simulink model "LGS_allFaultsSelected"  (R2019b)
settings: Solver=FixedStepDiscrete  StartTime=0.0  StopTime=45.0  FixedStep=0.1  RelTol=1e-3
model workspace (MAT data in the model file):
  fipData : object (value not decoded)
  fipName : object (value not decoded)
  stepSize = 0.1
undefined symbols (not defined in the file): ActualSystemCondition, ExpectedSystemBehavior, FailureCondition, FailureConditionObserver, LibFailureCondition
libraries: LibFaultInjectionControls x190, commrandsrc3 x70, simulink x3
(part 34 of 41)

== system LGS_allFaultsSelected/Gears/left gear cylinder/sensor locked retracted/FIP3/LG sensor locked retracted FIP3 ==
  In1 : Inport
  Commit Any Bool : Subsystem  mask(FailureMode){isActive=on, isDSF=off, FailureRate=1.0E-3, useDefaultMt_copy=off, MaintenanceTask=0, useDefaultMt=off, RiskTime=0, useDefaultRt=off, File=[], DSFjson=JSON}
      mask prompts: isActive "is Active"; isDSF "DSF Trigger"; useDefaultMt_copy "set"; useDefaultMt "set"; useDefaultRt "set"
      mask TypeOptions isActive: Trigger FIP/Active
      mask TypeOptions isDSF: Trigger FIP/isDSF
      mask Callback isDSF:
      | a = Simulink.Mask.get(gcb);
      | disp(a);
      | d = a.DialogControls();
      | disp(d);
      | for i = 1:size(d,2)
      |     if strcmp(d(i).Name, 'ParameterGroupVar')
      |         basicFip_ctrl = d(i).getDialogControl('BasicFipParam');
      |         dsFip_ctrl = d(i).getDialogControl('DSFipParam');
      | 
      |         if strcmp(get_param(gcb, 'isDSF'), 'on')
      | %            basicFip_ctrl.Visible = 'off';
      |             basicFip_ctrl.Enabled = 'off';
      | 
      |             dsFip_ctrl.Enabled = 'on';
      | %            dsFip_ctrl.Visible = 'on';
      |         else
      |             basicFip_ctrl.Enabled = 'on';
      | %            basicFip_ctrl.Visible = 'on';
      | 
      | %            dsFip_ctrl.Visible = 'off';
      |             dsFip_ctrl.Enabled = 'off';
      |         end
      |     end
      | end
      mask TypeOptions FailureRate: Trigger FIP/FailureRate
      mask Callback useDefaultMt_copy:
      | a = Simulink.Mask.get(gcb);
      | d = a.Parameters();
      | for i = 1:size(d,2)
      |     if strcmp(d(i).Name, 'MaintenanceTask')
      |         if strcmp(get_param(gcb, 'useDefaultMt'), 'off')
      |             set_param(gcb,'MaintenanceTask', '0')
      |             d(i).Enabled = 'off';
      |         else
      |             d(i).Enabled = 'on';
      |         end
      |     end
      | end
      mask TypeOptions MaintenanceTask: Trigger FIP/MaintenanceTask
      mask Callback useDefaultMt:
      | a = Simulink.Mask.get(gcb);
      | d = a.Parameters();
      | for i = 1:size(d,2)
      |     if strcmp(d(i).Name, 'MaintenanceTask')
      |         if strcmp(get_param(gcb, 'useDefaultMt'), 'off')
      |             set_param(gcb,'MaintenanceTask', '0')
      |             d(i).Enabled = 'off';
      |         else
      |             d(i).Enabled = 'on';
      |         end
      |     end
      | end
      mask TypeOptions RiskTime: Trigger FIP/RiskTime
      mask Callback useDefaultRt:
      | a = Simulink.Mask.get(gcb);
      | d = a.Parameters();
      | for i = 1:size(d,2)
      |     if strcmp(d(i).Name, 'RiskTime')
      |         if strcmp(get_param(gcb, 'useDefaultRt'), 'off')
      |             set_param(gcb,'RiskTime', '0')
      |             d(i).Enabled = 'off';
      |         else
      |             d(i).Enabled = 'on';
      |         end
      |     end
      | end
      mask TypeOptions DSFjson: Trigger FIP/DSFjson
      mask DialogControl DescGroupVar Prompt: Any Bool
      mask DialogControl DescTextVar Prompt: Controls for a fault with random boolean as result type
      mask DialogControl BasicFipBehavior Prompt: Failure Mode Behavior
      mask DialogControl BasicFipParamTab Prompt: Failure Mode Occurrence
      mask DialogControl BasicFipParam Prompt: Parameters
      mask DialogControl FailureRate_label Prompt: Failure Rate [1/h]
      mask DialogControl MaintenanceTask_label Prompt: Maintenance Task [h]
      mask DialogControl RiskTime_label Prompt: Risk time [h]
      mask DialogControl DSFipParamTab Prompt: Dependent System Information
      mask DialogControl DSFipParam Prompt: Parameters
      mask DialogControl LoadCSV Prompt: Browse
      mask DialogControl LoadCSV Callback:
      | [file,path,indx] = uigetfile('*.csv');
      | try
      |     set_param(gcb, 'File', append(path,file));
      |     file = fopen(append(path,file));
      | 
      |     fips = {};
      |     cutsets = {};
      | 
      |     line = fgetl(file);
      |     while ischar(line)
      |         disp(join([' > Processing: ',line]));
      |         splitString = split(line, ';');
      |         if isequal(splitString{1}, 'Cut set')
      |             disp('   > Found Cut set');
      |             cs = splitString(2:end-1);
      |             disp(cs);
      |             cutsets{end+1} = cs';
      |         else
      |             disp('   > Found FIP');
      |             if ~isequal("h", splitString(7))
      |                 disp('no time format except hour is supported');
      |             end
      |             fip = {};
      |             fip.id = splitString(1);
      |             fip.path = splitString(3);
      |             fip.rate = splitString(4);
      |             fip.checkInterval = splitString(6);
      |             disp(fip);
      |             fips{end+1} = fip;
      |         end
      |         line = fgetl(file);
      |     end
      | 
      |     fclose(file);
      | 
      |     DSF = {};
      |     DSF.fips = fips;
      |     DSF.cutsets = cutsets;
      | 
      |     VarCSText = jsonencode(DSF);
      |     set_param(gcb, 'DSFjson', VarCSText);
      | catch
      | end
  Permanently Blocked False : Subsystem  mask(FailureMode){isActive=on, isDSF=off, Value=false, FailureRate=1.0E-3, useDefaultMt_copy=off, MaintenanceTask=0, useDefaultMt=off, RiskTime=0, useDefaultRt=off, File=[], DSFjson=JSON}
      mask prompts: isActive "is Active"; isDSF "DSF Trigger"; Value "Bool Value"; useDefaultMt_copy "set"; useDefaultMt "set"; useDefaultRt "set"
      mask TypeOptions isActive: Trigger FIP/Active
      mask TypeOptions isDSF: Trigger FIP/isDSF
      mask Callback isDSF:
      | a = Simulink.Mask.get(gcb);
      | disp(a);
      | d = a.DialogControls();
      | disp(d);
      | for i = 1:size(d,2)
      |     if strcmp(d(i).Name, 'ParameterGroupVar')
      |         basicFip_ctrl = d(i).getDialogControl('BasicFipParam');
      |         dsFip_ctrl = d(i).getDialogControl('DSFipParam');
      | 
      |         if strcmp(get_param(gcb, 'isDSF'), 'on')
      | %            basicFip_ctrl.Visible = 'off';
      |             basicFip_ctrl.Enabled = 'off';
      | 
      |             dsFip_ctrl.Enabled = 'on';
      | %            dsFip_ctrl.Visible = 'on';
      |         else
      |             basicFip_ctrl.Enabled = 'on';
      | %            basicFip_ctrl.Visible = 'on';
      | 
      | %            dsFip_ctrl.Visible = 'off';
      |             dsFip_ctrl.Enabled = 'off';
      |         end
      |     end
      | end
      mask TypeOptions Value: CommitValue/Value
      mask TypeOptions FailureRate: Trigger FIP/FailureRate
      mask Callback useDefaultMt_copy:
      | a = Simulink.Mask.get(gcb);
      | d = a.Parameters();
      | for i = 1:size(d,2)
      |     if strcmp(d(i).Name, 'MaintenanceTask')
      |         if strcmp(get_param(gcb, 'useDefaultMt'), 'off')
      |             set_param(gcb,'MaintenanceTask', '0')
      |             d(i).Enabled = 'off';
      |         else
      |             d(i).Enabled = 'on';
      |         end
      |     end
      | end
      mask TypeOptions MaintenanceTask: Trigger FIP/MaintenanceTask
      mask Callback useDefaultMt:
      | a = Simulink.Mask.get(gcb);
      | d = a.Parameters();
      | for i = 1:size(d,2)
      |     if strcmp(d(i).Name, 'MaintenanceTask')
      |         if strcmp(get_param(gcb, 'useDefaultMt'), 'off')
      |             set_param(gcb,'MaintenanceTask', '0')
      |             d(i).Enabled = 'off';
      |         else
      |             d(i).Enabled = 'on';
      |         end
      |     end
      | end
      mask TypeOptions RiskTime: Trigger FIP/RiskTime
      mask Callback useDefaultRt:
      | a = Simulink.Mask.get(gcb);
      | d = a.Parameters();
      | for i = 1:size(d,2)
      |     if strcmp(d(i).Name, 'RiskTime')
      |         if strcmp(get_param(gcb, 'useDefaultRt'), 'off')
      |             set_param(gcb,'RiskTime', '0')
      |             d(i).Enabled = 'off';
      |         else
      |             d(i).Enabled = 'on';
      |         end
      |     end
      | end
      mask TypeOptions DSFjson: Trigger FIP/DSFjson
      mask DialogControl DescGroupVar Prompt: Bool
      mask DialogControl DescTextVar Prompt: Controls for a fault with boolean as result type
      mask DialogControl BasicFipBehavior Prompt: Failure Mode Behavior
      mask DialogControl BasicFipParamTab Prompt: Failure Mode Occurrence
      mask DialogControl BasicFipParam Prompt: Parameters
      mask DialogControl FailureRate_label Prompt: Failure Rate [1/h]
      mask DialogControl MaintenanceTask_label Prompt: Maintenance Task [h]
      mask DialogControl RiskTime_label Prompt: Risk time [h]
      mask DialogControl DSFipParamTab Prompt: Dependent System Information
      mask DialogControl DSFipParam Prompt: Parameters
      mask DialogControl LoadCSV Prompt: Browse
      mask DialogControl LoadCSV Callback:
      | [file,path,indx] = uigetfile('*.csv');
      | try
      |     set_param(gcb, 'File', append(path,file));
      |     file = fopen(append(path,file));
      | 
      |     fips = {};
      |     cutsets = {};
      | 
      |     line = fgetl(file);
      |     while ischar(line)
      |         disp(join([' > Processing: ',line]));
      |         splitString = split(line, ';');
      |         if isequal(splitString{1}, 'Cut set')
      |             disp('   > Found Cut set');
      |             cs = splitString(2:end-1);
      |             disp(cs);
      |             cutsets{end+1} = cs';
      |         else
      |             disp('   > Found FIP');
      |             if ~isequal("h", splitString(7))
      |                 disp('no time format except hour is supported');
      |             end
      |             fip = {};
      |             fip.id = splitString(1);
      |             fip.path = splitString(3);
      |             fip.rate = splitString(4);
      |             fip.checkInterval = splitString(6);
      |             disp(fip);
      |             fips{end+1} = fip;
      |         end
      |         line = fgetl(file);
      |     end
      | 
      |     fclose(file);
      | 
      |     DSF = {};
      |     DSF.fips = fips;
      |     DSF.cutsets = cutsets;
      | 
      |     VarCSText = jsonencode(DSF);
      |     set_param(gcb, 'DSFjson', VarCSText);
      | catch
      | end
  Permanently Blocked True : Subsystem  mask(FailureMode){isActive=on, isDSF=off, Value=true, FailureRate=1.0E-3, useDefaultMt_copy=off, MaintenanceTask=0, useDefaultMt=off, RiskTime=0, useDefaultRt=off, File=[], DSFjson=JSON}
      mask prompts: isActive "is Active"; isDSF "DSF Trigger"; Value "Bool Value"; useDefaultMt_copy "set"; useDefaultMt "set"; useDefaultRt "set"
      mask TypeOptions isActive: Trigger FIP/Active
      mask TypeOptions isDSF: Trigger FIP/isDSF
      mask Callback isDSF:
      | a = Simulink.Mask.get(gcb);
      | disp(a);
      | d = a.DialogControls();
      | disp(d);
      | for i = 1:size(d,2)
      |     if strcmp(d(i).Name, 'ParameterGroupVar')
      |         basicFip_ctrl = d(i).getDialogControl('BasicFipParam');
      |         dsFip_ctrl = d(i).getDialogControl('DSFipParam');
      | 
      |         if strcmp(get_param(gcb, 'isDSF'), 'on')
      | %            basicFip_ctrl.Visible = 'off';
      |             basicFip_ctrl.Enabled = 'off';
      | 
      |             dsFip_ctrl.Enabled = 'on';
      | %            dsFip_ctrl.Visible = 'on';
      |         else
      |             basicFip_ctrl.Enabled = 'on';
      | %            basicFip_ctrl.Visible = 'on';
      | 
      | %            dsFip_ctrl.Visible = 'off';
      |             dsFip_ctrl.Enabled = 'off';
      |         end
      |     end
      | end
      mask TypeOptions Value: CommitValue/Value
      mask TypeOptions FailureRate: Trigger FIP/FailureRate
      mask Callback useDefaultMt_copy:
      | a = Simulink.Mask.get(gcb);
      | d = a.Parameters();
      | for i = 1:size(d,2)
      |     if strcmp(d(i).Name, 'MaintenanceTask')
      |         if strcmp(get_param(gcb, 'useDefaultMt'), 'off')
      |             set_param(gcb,'MaintenanceTask', '0')
      |             d(i).Enabled = 'off';
      |         else
      |             d(i).Enabled = 'on';
      |         end
      |     end
      | end
      mask TypeOptions MaintenanceTask: Trigger FIP/MaintenanceTask
      mask Callback useDefaultMt:
      | a = Simulink.Mask.get(gcb);
      | d = a.Parameters();
      | for i = 1:size(d,2)
      |     if strcmp(d(i).Name, 'MaintenanceTask')
      |         if strcmp(get_param(gcb, 'useDefaultMt'), 'off')
      |             set_param(gcb,'MaintenanceTask', '0')
      |             d(i).Enabled = 'off';
      |         else
      |             d(i).Enabled = 'on';
      |         end
      |     end
      | end
      mask TypeOptions RiskTime: Trigger FIP/RiskTime
      mask Callback useDefaultRt:
      | a = Simulink.Mask.get(gcb);
      | d = a.Parameters();
      | for i = 1:size(d,2)
      |     if strcmp(d(i).Name, 'RiskTime')
      |         if strcmp(get_param(gcb, 'useDefaultRt'), 'off')
      |             set_param(gcb,'RiskTime', '0')
      |             d(i).Enabled = 'off';
      |         else
      |             d(i).Enabled = 'on';
      |         end
      |     end
      | end
      mask TypeOptions DSFjson: Trigger FIP/DSFjson
      mask DialogControl DescGroupVar Prompt: Bool
      mask DialogControl DescTextVar Prompt: Controls for a fault with boolean as result type
      mask DialogControl BasicFipBehavior Prompt: Failure Mode Behavior
      mask DialogControl BasicFipParamTab Prompt: Failure Mode Occurrence
      mask DialogControl BasicFipParam Prompt: Parameters
      mask DialogControl FailureRate_label Prompt: Failure Rate [1/h]
      mask DialogControl MaintenanceTask_label Prompt: Maintenance Task [h]
      mask DialogControl RiskTime_label Prompt: Risk time [h]
      mask DialogControl DSFipParamTab Prompt: Dependent System Information
      mask DialogControl DSFipParam Prompt: Parameters
      mask DialogControl LoadCSV Prompt: Browse
      mask DialogControl LoadCSV Callback:
      | [file,path,indx] = uigetfile('*.csv');
      | try
      |     set_param(gcb, 'File', append(path,file));
      |     file = fopen(append(path,file));
      | 
      |     fips = {};
      |     cutsets = {};
      | 
      |     line = fgetl(file);
      |     while ischar(line)
      |         disp(join([' > Processing: ',line]));
      |         splitString = split(line, ';');
      |         if isequal(splitString{1}, 'Cut set')
      |             disp('   > Found Cut set');
      |             cs = splitString(2:end-1);
      |             disp(cs);
      |             cutsets{end+1} = cs';
      |         else
      |             disp('   > Found FIP');
      |             if ~isequal("h", splitString(7))
      |                 disp('no time format except hour is supported');
      |             end
      |             fip = {};
      |             fip.id = splitString(1);
      |             fip.path = splitString(3);
      |             fip.rate = splitString(4);
      |             fip.checkInterval = splitString(6);
      |             disp(fip);
      |             fips{end+1} = fip;
      |         end
      |         line = fgetl(file);
      |     end
      | 
      |     fclose(file);
      | 
      |     DSF = {};
      |     DSF.fips = fips;
      |     DSF.cutsets = cutsets;
      | 
      |     VarCSText = jsonencode(DSF);
      |     set_param(gcb, 'DSFjson', VarCSText);
      | catch
      | end
  Out1 : Outport
  wires:
  In1/1 -> Permanently Blocked True/1(In1)
  Commit Any Bool/1(Out1) -> Out1/1
  Permanently Blocked False/1(Out1) -> Commit Any Bool/1(In1)
  Permanently Blocked True/1(Out1) -> Permanently Blocked False/1(In1)

== system LGS_allFaultsSelected/Gears/right gear cylinder/sensor locked extended/FIP1/RG sensor locked extended FIP1 ==
  In1 : Inport
  Commit Any Bool : Subsystem  mask(FailureMode){isActive=on, isDSF=off, FailureRate=1.0E-3, useDefaultMt_copy=off, MaintenanceTask=0, useDefaultMt=off, RiskTime=0, useDefaultRt=off, File=[], DSFjson=JSON}
      mask prompts: isActive "is Active"; isDSF "DSF Trigger"; useDefaultMt_copy "set"; useDefaultMt "set"; useDefaultRt "set"
      mask TypeOptions isActive: Trigger FIP/Active
      mask TypeOptions isDSF: Trigger FIP/isDSF
      mask Callback isDSF:
      | a = Simulink.Mask.get(gcb);
      | disp(a);
      | d = a.DialogControls();
      | disp(d);
      | for i = 1:size(d,2)
      |     if strcmp(d(i).Name, 'ParameterGroupVar')
      |         basicFip_ctrl = d(i).getDialogControl('BasicFipParam');
      |         dsFip_ctrl = d(i).getDialogControl('DSFipParam');
      | 
      |         if strcmp(get_param(gcb, 'isDSF'), 'on')
      | %            basicFip_ctrl.Visible = 'off';
      |             basicFip_ctrl.Enabled = 'off';
      | 
      |             dsFip_ctrl.Enabled = 'on';
      | %            dsFip_ctrl.Visible = 'on';
      |         else
      |             basicFip_ctrl.Enabled = 'on';
      | %            basicFip_ctrl.Visible = 'on';
      | 
      | %            dsFip_ctrl.Visible = 'off';
      |             dsFip_ctrl.Enabled = 'off';
      |         end
      |     end
      | end
      mask TypeOptions FailureRate: Trigger FIP/FailureRate
      mask Callback useDefaultMt_copy:
      | a = Simulink.Mask.get(gcb);
      | d = a.Parameters();
      | for i = 1:size(d,2)
      |     if strcmp(d(i).Name, 'MaintenanceTask')
      |         if strcmp(get_param(gcb, 'useDefaultMt'), 'off')
      |             set_param(gcb,'MaintenanceTask', '0')
      |             d(i).Enabled = 'off';
      |         else
      |             d(i).Enabled = 'on';
      |         end
      |     end
      | end
      mask TypeOptions MaintenanceTask: Trigger FIP/MaintenanceTask
      mask Callback useDefaultMt:
      | a = Simulink.Mask.get(gcb);
      | d = a.Parameters();
      | for i = 1:size(d,2)
      |     if strcmp(d(i).Name, 'MaintenanceTask')
      |         if strcmp(get_param(gcb, 'useDefaultMt'), 'off')
      |             set_param(gcb,'MaintenanceTask', '0')
      |             d(i).Enabled = 'off';
      |         else
      |             d(i).Enabled = 'on';
      |         end
      |     end
      | end
      mask TypeOptions RiskTime: Trigger FIP/RiskTime
      mask Callback useDefaultRt:
      | a = Simulink.Mask.get(gcb);
      | d = a.Parameters();
      | for i = 1:size(d,2)
      |     if strcmp(d(i).Name, 'RiskTime')
      |         if strcmp(get_param(gcb, 'useDefaultRt'), 'off')
      |             set_param(gcb,'RiskTime', '0')
      |             d(i).Enabled = 'off';
      |         else
      |             d(i).Enabled = 'on';
      |         end
      |     end
      | end
      mask TypeOptions DSFjson: Trigger FIP/DSFjson
      mask DialogControl DescGroupVar Prompt: Any Bool
      mask DialogControl DescTextVar Prompt: Controls for a fault with random boolean as result type
      mask DialogControl BasicFipBehavior Prompt: Failure Mode Behavior
      mask DialogControl BasicFipParamTab Prompt: Failure Mode Occurrence
      mask DialogControl BasicFipParam Prompt: Parameters
      mask DialogControl FailureRate_label Prompt: Failure Rate [1/h]
      mask DialogControl MaintenanceTask_label Prompt: Maintenance Task [h]
      mask DialogControl RiskTime_label Prompt: Risk time [h]
      mask DialogControl DSFipParamTab Prompt: Dependent System Information
      mask DialogControl DSFipParam Prompt: Parameters
      mask DialogControl LoadCSV Prompt: Browse
      mask DialogControl LoadCSV Callback:
      | [file,path,indx] = uigetfile('*.csv');
      | try
      |     set_param(gcb, 'File', append(path,file));
      |     file = fopen(append(path,file));
      | 
      |     fips = {};
      |     cutsets = {};
      | 
      |     line = fgetl(file);
      |     while ischar(line)
      |         disp(join([' > Processing: ',line]));
      |         splitString = split(line, ';');
      |         if isequal(splitString{1}, 'Cut set')
      |             disp('   > Found Cut set');
      |             cs = splitString(2:end-1);
      |             disp(cs);
      |             cutsets{end+1} = cs';
      |         else
      |             disp('   > Found FIP');
      |             if ~isequal("h", splitString(7))
      |                 disp('no time format except hour is supported');
      |             end
      |             fip = {};
      |             fip.id = splitString(1);
      |             fip.path = splitString(3);
      |             fip.rate = splitString(4);
      |             fip.checkInterval = splitString(6);
      |             disp(fip);
      |             fips{end+1} = fip;
      |         end
      |         line = fgetl(file);
      |     end
      | 
      |     fclose(file);
      | 
      |     DSF = {};
      |     DSF.fips = fips;
      |     DSF.cutsets = cutsets;
      | 
      |     VarCSText = jsonencode(DSF);
      |     set_param(gcb, 'DSFjson', VarCSText);
      | catch
      | end
  Permanently Blocked False : Subsystem  mask(FailureMode){isActive=on, isDSF=off, Value=false, FailureRate=1.0E-3, useDefaultMt_copy=off, MaintenanceTask=0, useDefaultMt=off, RiskTime=0, useDefaultRt=off, File=[], DSFjson=JSON}
      mask prompts: isActive "is Active"; isDSF "DSF Trigger"; Value "Bool Value"; useDefaultMt_copy "set"; useDefaultMt "set"; useDefaultRt "set"
      mask TypeOptions isActive: Trigger FIP/Active
      mask TypeOptions isDSF: Trigger FIP/isDSF
      mask Callback isDSF:
      | a = Simulink.Mask.get(gcb);
      | disp(a);
      | d = a.DialogControls();
      | disp(d);
      | for i = 1:size(d,2)
      |     if strcmp(d(i).Name, 'ParameterGroupVar')
      |         basicFip_ctrl = d(i).getDialogControl('BasicFipParam');
      |         dsFip_ctrl = d(i).getDialogControl('DSFipParam');
      | 
      |         if strcmp(get_param(gcb, 'isDSF'), 'on')
      | %            basicFip_ctrl.Visible = 'off';
      |             basicFip_ctrl.Enabled = 'off';
      | 
      |             dsFip_ctrl.Enabled = 'on';
      | %            dsFip_ctrl.Visible = 'on';
      |         else
      |             basicFip_ctrl.Enabled = 'on';
      | %            basicFip_ctrl.Visible = 'on';
      | 
      | %            dsFip_ctrl.Visible = 'off';
      |             dsFip_ctrl.Enabled = 'off';
      |         end
      |     end
      | end
      mask TypeOptions Value: CommitValue/Value
      mask TypeOptions FailureRate: Trigger FIP/FailureRate
      mask Callback useDefaultMt_copy:
      | a = Simulink.Mask.get(gcb);
      | d = a.Parameters();
      | for i = 1:size(d,2)
      |     if strcmp(d(i).Name, 'MaintenanceTask')
      |         if strcmp(get_param(gcb, 'useDefaultMt'), 'off')
      |             set_param(gcb,'MaintenanceTask', '0')
      |             d(i).Enabled = 'off';
      |         else
      |             d(i).Enabled = 'on';
      |         end
      |     end
      | end
      mask TypeOptions MaintenanceTask: Trigger FIP/MaintenanceTask
      mask Callback useDefaultMt:
      | a = Simulink.Mask.get(gcb);
      | d = a.Parameters();
      | for i = 1:size(d,2)
      |     if strcmp(d(i).Name, 'MaintenanceTask')
      |         if strcmp(get_param(gcb, 'useDefaultMt'), 'off')
      |             set_param(gcb,'MaintenanceTask', '0')
      |             d(i).Enabled = 'off';
      |         else
      |             d(i).Enabled = 'on';
      |         end
      |     end
      | end
      mask TypeOptions RiskTime: Trigger FIP/RiskTime
      mask Callback useDefaultRt:
      | a = Simulink.Mask.get(gcb);
      | d = a.Parameters();
      | for i = 1:size(d,2)
      |     if strcmp(d(i).Name, 'RiskTime')
      |         if strcmp(get_param(gcb, 'useDefaultRt'), 'off')
      |             set_param(gcb,'RiskTime', '0')
      |             d(i).Enabled = 'off';
      |         else
      |             d(i).Enabled = 'on';
      |         end
      |     end
      | end
      mask TypeOptions DSFjson: Trigger FIP/DSFjson
      mask DialogControl DescGroupVar Prompt: Bool
      mask DialogControl DescTextVar Prompt: Controls for a fault with boolean as result type
      mask DialogControl BasicFipBehavior Prompt: Failure Mode Behavior
      mask DialogControl BasicFipParamTab Prompt: Failure Mode Occurrence
      mask DialogControl BasicFipParam Prompt: Parameters
      mask DialogControl FailureRate_label Prompt: Failure Rate [1/h]
      mask DialogControl MaintenanceTask_label Prompt: Maintenance Task [h]
      mask DialogControl RiskTime_label Prompt: Risk time [h]
      mask DialogControl DSFipParamTab Prompt: Dependent System Information
      mask DialogControl DSFipParam Prompt: Parameters
      mask DialogControl LoadCSV Prompt: Browse
      mask DialogControl LoadCSV Callback:
      | [file,path,indx] = uigetfile('*.csv');
      | try
      |     set_param(gcb, 'File', append(path,file));
      |     file = fopen(append(path,file));
      | 
      |     fips = {};
      |     cutsets = {};
      | 
      |     line = fgetl(file);
      |     while ischar(line)
      |         disp(join([' > Processing: ',line]));
      |         splitString = split(line, ';');
      |         if isequal(splitString{1}, 'Cut set')
      |             disp('   > Found Cut set');
      |             cs = splitString(2:end-1);
      |             disp(cs);
      |             cutsets{end+1} = cs';
      |         else
      |             disp('   > Found FIP');
      |             if ~isequal("h", splitString(7))
      |                 disp('no time format except hour is supported');
      |             end
      |             fip = {};
      |             fip.id = splitString(1);
      |             fip.path = splitString(3);
      |             fip.rate = splitString(4);
      |             fip.checkInterval = splitString(6);
      |             disp(fip);
      |             fips{end+1} = fip;
      |         end
      |         line = fgetl(file);
      |     end
      | 
      |     fclose(file);
      | 
      |     DSF = {};
      |     DSF.fips = fips;
      |     DSF.cutsets = cutsets;
      | 
      |     VarCSText = jsonencode(DSF);
      |     set_param(gcb, 'DSFjson', VarCSText);
      | catch
      | end
  Permanently Blocked True : Subsystem  mask(FailureMode){isActive=on, isDSF=off, Value=true, FailureRate=1.0E-3, useDefaultMt_copy=off, MaintenanceTask=0, useDefaultMt=off, RiskTime=0, useDefaultRt=off, File=[], DSFjson=JSON}
      mask prompts: isActive "is Active"; isDSF "DSF Trigger"; Value "Bool Value"; useDefaultMt_copy "set"; useDefaultMt "set"; useDefaultRt "set"
      mask TypeOptions isActive: Trigger FIP/Active
      mask TypeOptions isDSF: Trigger FIP/isDSF
      mask Callback isDSF:
      | a = Simulink.Mask.get(gcb);
      | disp(a);
      | d = a.DialogControls();
      | disp(d);
      | for i = 1:size(d,2)
      |     if strcmp(d(i).Name, 'ParameterGroupVar')
      |         basicFip_ctrl = d(i).getDialogControl('BasicFipParam');
      |         dsFip_ctrl = d(i).getDialogControl('DSFipParam');
      | 
      |         if strcmp(get_param(gcb, 'isDSF'), 'on')
      | %            basicFip_ctrl.Visible = 'off';
      |             basicFip_ctrl.Enabled = 'off';
      | 
      |             dsFip_ctrl.Enabled = 'on';
      | %            dsFip_ctrl.Visible = 'on';
      |         else
      |             basicFip_ctrl.Enabled = 'on';
      | %            basicFip_ctrl.Visible = 'on';
      | 
      | %            dsFip_ctrl.Visible = 'off';
      |             dsFip_ctrl.Enabled = 'off';
      |         end
      |     end
      | end
      mask TypeOptions Value: CommitValue/Value
      mask TypeOptions FailureRate: Trigger FIP/FailureRate
      mask Callback useDefaultMt_copy:
      | a = Simulink.Mask.get(gcb);
      | d = a.Parameters();
      | for i = 1:size(d,2)
      |     if strcmp(d(i).Name, 'MaintenanceTask')
      |         if strcmp(get_param(gcb, 'useDefaultMt'), 'off')
      |             set_param(gcb,'MaintenanceTask', '0')
      |             d(i).Enabled = 'off';
      |         else
      |             d(i).Enabled = 'on';
      |         end
      |     end
      | end
      mask TypeOptions MaintenanceTask: Trigger FIP/MaintenanceTask
      mask Callback useDefaultMt:
      | a = Simulink.Mask.get(gcb);
      | d = a.Parameters();
      | for i = 1:size(d,2)
      |     if strcmp(d(i).Name, 'MaintenanceTask')
      |         if strcmp(get_param(gcb, 'useDefaultMt'), 'off')
      |             set_param(gcb,'MaintenanceTask', '0')
      |             d(i).Enabled = 'off';
      |         else
      |             d(i).Enabled = 'on';
      |         end
      |     end
      | end
      mask TypeOptions RiskTime: Trigger FIP/RiskTime
      mask Callback useDefaultRt:
      | a = Simulink.Mask.get(gcb);
      | d = a.Parameters();
      | for i = 1:size(d,2)
      |     if strcmp(d(i).Name, 'RiskTime')
      |         if strcmp(get_param(gcb, 'useDefaultRt'), 'off')
      |             set_param(gcb,'RiskTime', '0')
      |             d(i).Enabled = 'off';
      |         else
      |             d(i).Enabled = 'on';
      |         end
      |     end
      | end
      mask TypeOptions DSFjson: Trigger FIP/DSFjson
      mask DialogControl DescGroupVar Prompt: Bool
      mask DialogControl DescTextVar Prompt: Controls for a fault with boolean as result type
      mask DialogControl BasicFipBehavior Prompt: Failure Mode Behavior
      mask DialogControl BasicFipParamTab Prompt: Failure Mode Occurrence
      mask DialogControl BasicFipParam Prompt: Parameters
      mask DialogControl FailureRate_label Prompt: Failure Rate [1/h]
      mask DialogControl MaintenanceTask_label Prompt: Maintenance Task [h]
      mask DialogControl RiskTime_label Prompt: Risk time [h]
      mask DialogControl DSFipParamTab Prompt: Dependent System Information
      mask DialogControl DSFipParam Prompt: Parameters
      mask DialogControl LoadCSV Prompt: Browse
      mask DialogControl LoadCSV Callback:
      | [file,path,indx] = uigetfile('*.csv');
      | try
      |     set_param(gcb, 'File', append(path,file));
      |     file = fopen(append(path,file));
      | 
      |     fips = {};
      |     cutsets = {};
      | 
      |     line = fgetl(file);
      |     while ischar(line)
      |         disp(join([' > Processing: ',line]));
      |         splitString = split(line, ';');
      |         if isequal(splitString{1}, 'Cut set')
      |             disp('   > Found Cut set');
      |             cs = splitString(2:end-1);
      |             disp(cs);
      |             cutsets{end+1} = cs';
      |         else
      |             disp('   > Found FIP');
      |             if ~isequal("h", splitString(7))
      |                 disp('no time format except hour is supported');
      |             end
      |             fip = {};
      |             fip.id = splitString(1);
      |             fip.path = splitString(3);
      |             fip.rate = splitString(4);
      |             fip.checkInterval = splitString(6);
      |             disp(fip);
      |             fips{end+1} = fip;
      |         end
      |         line = fgetl(file);
      |     end
      | 
      |     fclose(file);
      | 
      |     DSF = {};
      |     DSF.fips = fips;
      |     DSF.cutsets = cutsets;
      | 
      |     VarCSText = jsonencode(DSF);
      |     set_param(gcb, 'DSFjson', VarCSText);
      | catch
      | end
  Out1 : Outport
  wires:
  In1/1 -> Permanently Blocked True/1(In1)
  Commit Any Bool/1(Out1) -> Out1/1
  Permanently Blocked False/1(Out1) -> Commit Any Bool/1(In1)
  Permanently Blocked True/1(Out1) -> Permanently Blocked False/1(In1)

== system LGS_allFaultsSelected/Gears/right gear cylinder/sensor locked extended/FIP2/RG sensor locked extended FIP2 ==
  In1 : Inport
  Commit Any Bool : Subsystem  mask(FailureMode){isActive=on, isDSF=off, FailureRate=1.0E-3, useDefaultMt_copy=off, MaintenanceTask=0, useDefaultMt=off, RiskTime=0, useDefaultRt=off, File=[], DSFjson=JSON}
      mask prompts: isActive "is Active"; isDSF "DSF Trigger"; useDefaultMt_copy "set"; useDefaultMt "set"; useDefaultRt "set"
      mask TypeOptions isActive: Trigger FIP/Active
      mask TypeOptions isDSF: Trigger FIP/isDSF
      mask Callback isDSF:
      | a = Simulink.Mask.get(gcb);
      | disp(a);
      | d = a.DialogControls();
      | disp(d);
      | for i = 1:size(d,2)
      |     if strcmp(d(i).Name, 'ParameterGroupVar')
      |         basicFip_ctrl = d(i).getDialogControl('BasicFipParam');
      |         dsFip_ctrl = d(i).getDialogControl('DSFipParam');
      | 
      |         if strcmp(get_param(gcb, 'isDSF'), 'on')
      | %            basicFip_ctrl.Visible = 'off';
      |             basicFip_ctrl.Enabled = 'off';
      | 
      |             dsFip_ctrl.Enabled = 'on';
      | %            dsFip_ctrl.Visible = 'on';
      |         else
      |             basicFip_ctrl.Enabled = 'on';
      | %            basicFip_ctrl.Visible = 'on';
      | 
      | %            dsFip_ctrl.Visible = 'off';
      |             dsFip_ctrl.Enabled = 'off';
      |         end
      |     end
      | end
      mask TypeOptions FailureRate: Trigger FIP/FailureRate
      mask Callback useDefaultMt_copy:
      | a = Simulink.Mask.get(gcb);
      | d = a.Parameters();
      | for i = 1:size(d,2)
      |     if strcmp(d(i).Name, 'MaintenanceTask')
      |         if strcmp(get_param(gcb, 'useDefaultMt'), 'off')
      |             set_param(gcb,'MaintenanceTask', '0')
      |             d(i).Enabled = 'off';
      |         else
      |             d(i).Enabled = 'on';
      |         end
      |     end
      | end
      mask TypeOptions MaintenanceTask: Trigger FIP/MaintenanceTask
      mask Callback useDefaultMt:
      | a = Simulink.Mask.get(gcb);
      | d = a.Parameters();
      | for i = 1:size(d,2)
      |     if strcmp(d(i).Name, 'MaintenanceTask')
      |         if strcmp(get_param(gcb, 'useDefaultMt'), 'off')
      |             set_param(gcb,'MaintenanceTask', '0')
      |             d(i).Enabled = 'off';
      |         else
      |             d(i).Enabled = 'on';
      |         end
      |     end
      | end
      mask TypeOptions RiskTime: Trigger FIP/RiskTime
      mask Callback useDefaultRt:
      | a = Simulink.Mask.get(gcb);
      | d = a.Parameters();
      | for i = 1:size(d,2)
      |     if strcmp(d(i).Name, 'RiskTime')
      |         if strcmp(get_param(gcb, 'useDefaultRt'), 'off')
      |             set_param(gcb,'RiskTime', '0')
      |             d(i).Enabled = 'off';
      |         else
      |             d(i).Enabled = 'on';
      |         end
      |     end
      | end
      mask TypeOptions DSFjson: Trigger FIP/DSFjson
      mask DialogControl DescGroupVar Prompt: Any Bool
      mask DialogControl DescTextVar Prompt: Controls for a fault with random boolean as result type
      mask DialogControl BasicFipBehavior Prompt: Failure Mode Behavior
      mask DialogControl BasicFipParamTab Prompt: Failure Mode Occurrence
      mask DialogControl BasicFipParam Prompt: Parameters
      mask DialogControl FailureRate_label Prompt: Failure Rate [1/h]
      mask DialogControl MaintenanceTask_label Prompt: Maintenance Task [h]
      mask DialogControl RiskTime_label Prompt: Risk time [h]
      mask DialogControl DSFipParamTab Prompt: Dependent System Information
      mask DialogControl DSFipParam Prompt: Parameters
      mask DialogControl LoadCSV Prompt: Browse
      mask DialogControl LoadCSV Callback:
      | [file,path,indx] = uigetfile('*.csv');
      | try
      |     set_param(gcb, 'File', append(path,file));
      |     file = fopen(append(path,file));
      | 
      |     fips = {};
      |     cutsets = {};
      | 
      |     line = fgetl(file);
      |     while ischar(line)
      |         disp(join([' > Processing: ',line]));
      |         splitString = split(line, ';');
      |         if isequal(splitString{1}, 'Cut set')
      |             disp('   > Found Cut set');
      |             cs = splitString(2:end-1);
      |             disp(cs);
      |             cutsets{end+1} = cs';
      |         else
      |             disp('   > Found FIP');
      |             if ~isequal("h", splitString(7))
      |                 disp('no time format except hour is supported');
      |             end
      |             fip = {};
      |             fip.id = splitString(1);
      |             fip.path = splitString(3);
      |             fip.rate = splitString(4);
      |             fip.checkInterval = splitString(6);
      |             disp(fip);
      |             fips{end+1} = fip;
      |         end
      |         line = fgetl(file);
      |     end
      | 
      |     fclose(file);
      | 
      |     DSF = {};
      |     DSF.fips = fips;
      |     DSF.cutsets = cutsets;
      | 
      |     VarCSText = jsonencode(DSF);
      |     set_param(gcb, 'DSFjson', VarCSText);
      | catch
      | end
  Permanently Blocked False : Subsystem  mask(FailureMode){isActive=on, isDSF=off, Value=false, FailureRate=1.0E-3, useDefaultMt_copy=off, MaintenanceTask=0, useDefaultMt=off, RiskTime=0, useDefaultRt=off, File=[], DSFjson=JSON}
      mask prompts: isActive "is Active"; isDSF "DSF Trigger"; Value "Bool Value"; useDefaultMt_copy "set"; useDefaultMt "set"; useDefaultRt "set"
      mask TypeOptions isActive: Trigger FIP/Active
      mask TypeOptions isDSF: Trigger FIP/isDSF
      mask Callback isDSF:
      | a = Simulink.Mask.get(gcb);
      | disp(a);
      | d = a.DialogControls();
      | disp(d);
      | for i = 1:size(d,2)
      |     if strcmp(d(i).Name, 'ParameterGroupVar')
      |         basicFip_ctrl = d(i).getDialogControl('BasicFipParam');
      |         dsFip_ctrl = d(i).getDialogControl('DSFipParam');
      | 
      |         if strcmp(get_param(gcb, 'isDSF'), 'on')
      | %            basicFip_ctrl.Visible = 'off';
      |             basicFip_ctrl.Enabled = 'off';
      | 
      |             dsFip_ctrl.Enabled = 'on';
      | %            dsFip_ctrl.Visible = 'on';
      |         else
      |             basicFip_ctrl.Enabled = 'on';
      | %            basicFip_ctrl.Visible = 'on';
      | 
      | %            dsFip_ctrl.Visible = 'off';
      |             dsFip_ctrl.Enabled = 'off';
      |         end
      |     end
      | end
      mask TypeOptions Value: CommitValue/Value
      mask TypeOptions FailureRate: Trigger FIP/FailureRate
      mask Callback useDefaultMt_copy:
      | a = Simulink.Mask.get(gcb);
      | d = a.Parameters();
      | for i = 1:size(d,2)
      |     if strcmp(d(i).Name, 'MaintenanceTask')
      |         if strcmp(get_param(gcb, 'useDefaultMt'), 'off')
      |             set_param(gcb,'MaintenanceTask', '0')
      |             d(i).Enabled = 'off';
      |         else
      |             d(i).Enabled = 'on';
      |         end
      |     end
      | end
      mask TypeOptions MaintenanceTask: Trigger FIP/MaintenanceTask
      mask Callback useDefaultMt:
      | a = Simulink.Mask.get(gcb);
      | d = a.Parameters();
      | for i = 1:size(d,2)
      |     if strcmp(d(i).Name, 'MaintenanceTask')
      |         if strcmp(get_param(gcb, 'useDefaultMt'), 'off')
      |             set_param(gcb,'MaintenanceTask', '0')
      |             d(i).Enabled = 'off';
      |         else
      |             d(i).Enabled = 'on';
      |         end
      |     end
      | end
      mask TypeOptions RiskTime: Trigger FIP/RiskTime
      mask Callback useDefaultRt:
      | a = Simulink.Mask.get(gcb);
      | d = a.Parameters();
      | for i = 1:size(d,2)
      |     if strcmp(d(i).Name, 'RiskTime')
      |         if strcmp(get_param(gcb, 'useDefaultRt'), 'off')
      |             set_param(gcb,'RiskTime', '0')
      |             d(i).Enabled = 'off';
      |         else
      |             d(i).Enabled = 'on';
      |         end
      |     end
      | end
      mask TypeOptions DSFjson: Trigger FIP/DSFjson
      mask DialogControl DescGroupVar Prompt: Bool
      mask DialogControl DescTextVar Prompt: Controls for a fault with boolean as result type
      mask DialogControl BasicFipBehavior Prompt: Failure Mode Behavior
      mask DialogControl BasicFipParamTab Prompt: Failure Mode Occurrence
      mask DialogControl BasicFipParam Prompt: Parameters
      mask DialogControl FailureRate_label Prompt: Failure Rate [1/h]
      mask DialogControl MaintenanceTask_label Prompt: Maintenance Task [h]
      mask DialogControl RiskTime_label Prompt: Risk time [h]
      mask DialogControl DSFipParamTab Prompt: Dependent System Information
      mask DialogControl DSFipParam Prompt: Parameters
      mask DialogControl LoadCSV Prompt: Browse
      mask DialogControl LoadCSV Callback:
      | [file,path,indx] = uigetfile('*.csv');
      | try
      |     set_param(gcb, 'File', append(path,file));
      |     file = fopen(append(path,file));
      | 
      |     fips = {};
      |     cutsets = {};
      | 
      |     line = fgetl(file);
      |     while ischar(line)
      |         disp(join([' > Processing: ',line]));
      |         splitString = split(line, ';');
      |         if isequal(splitString{1}, 'Cut set')
      |             disp('   > Found Cut set');
      |             cs = splitString(2:end-1);
      |             disp(cs);
      |             cutsets{end+1} = cs';
      |         else
      |             disp('   > Found FIP');
      |             if ~isequal("h", splitString(7))
      |                 disp('no time format except hour is supported');
      |             end
      |             fip = {};
      |             fip.id = splitString(1);
      |             fip.path = splitString(3);
      |             fip.rate = splitString(4);
      |             fip.checkInterval = splitString(6);
      |             disp(fip);
      |             fips{end+1} = fip;
      |         end
      |         line = fgetl(file);
      |     end
      | 
      |     fclose(file);
      | 
      |     DSF = {};
      |     DSF.fips = fips;
      |     DSF.cutsets = cutsets;
      | 
      |     VarCSText = jsonencode(DSF);
      |     set_param(gcb, 'DSFjson', VarCSText);
      | catch
      | end
  Permanently Blocked True : Subsystem  mask(FailureMode){isActive=on, isDSF=off, Value=true, FailureRate=1.0E-3, useDefaultMt_copy=off, MaintenanceTask=0, useDefaultMt=off, RiskTime=0, useDefaultRt=off, File=[], DSFjson=JSON}
      mask prompts: isActive "is Active"; isDSF "DSF Trigger"; Value "Bool Value"; useDefaultMt_copy "set"; useDefaultMt "set"; useDefaultRt "set"
      mask TypeOptions isActive: Trigger FIP/Active
      mask TypeOptions isDSF: Trigger FIP/isDSF
      mask Callback isDSF:
      | a = Simulink.Mask.get(gcb);
      | disp(a);
      | d = a.DialogControls();
      | disp(d);
      | for i = 1:size(d,2)
      |     if strcmp(d(i).Name, 'ParameterGroupVar')
      |         basicFip_ctrl = d(i).getDialogControl('BasicFipParam');
      |         dsFip_ctrl = d(i).getDialogControl('DSFipParam');
      | 
      |         if strcmp(get_param(gcb, 'isDSF'), 'on')
      | %            basicFip_ctrl.Visible = 'off';
      |             basicFip_ctrl.Enabled = 'off';
      | 
      |             dsFip_ctrl.Enabled = 'on';
      | %            dsFip_ctrl.Visible = 'on';
      |         else
      |             basicFip_ctrl.Enabled = 'on';
      | %            basicFip_ctrl.Visible = 'on';
      | 
      | %            dsFip_ctrl.Visible = 'off';
      |             dsFip_ctrl.Enabled = 'off';
      |         end
      |     end
      | end
      mask TypeOptions Value: CommitValue/Value
      mask TypeOptions FailureRate: Trigger FIP/FailureRate
      mask Callback useDefaultMt_copy:
      | a = Simulink.Mask.get(gcb);
      | d = a.Parameters();
      | for i = 1:size(d,2)
      |     if strcmp(d(i).Name, 'MaintenanceTask')
      |         if strcmp(get_param(gcb, 'useDefaultMt'), 'off')
      |             set_param(gcb,'MaintenanceTask', '0')
      |             d(i).Enabled = 'off';
      |         else
      |             d(i).Enabled = 'on';
      |         end
      |     end
      | end
      mask TypeOptions MaintenanceTask: Trigger FIP/MaintenanceTask
      mask Callback useDefaultMt:
      | a = Simulink.Mask.get(gcb);
      | d = a.Parameters();
      | for i = 1:size(d,2)
      |     if strcmp(d(i).Name, 'MaintenanceTask')
      |         if strcmp(get_param(gcb, 'useDefaultMt'), 'off')
      |             set_param(gcb,'MaintenanceTask', '0')
      |             d(i).Enabled = 'off';
      |         else
      |             d(i).Enabled = 'on';
      |         end
      |     end
      | end
      mask TypeOptions RiskTime: Trigger FIP/RiskTime
      mask Callback useDefaultRt:
      | a = Simulink.Mask.get(gcb);
      | d = a.Parameters();
      | for i = 1:size(d,2)
      |     if strcmp(d(i).Name, 'RiskTime')
      |         if strcmp(get_param(gcb, 'useDefaultRt'), 'off')
      |             set_param(gcb,'RiskTime', '0')
      |             d(i).Enabled = 'off';
      |         else
      |             d(i).Enabled = 'on';
      |         end
      |     end
      | end
      mask TypeOptions DSFjson: Trigger FIP/DSFjson
      mask DialogControl DescGroupVar Prompt: Bool
      mask DialogControl DescTextVar Prompt: Controls for a fault with boolean as result type
      mask DialogControl BasicFipBehavior Prompt: Failure Mode Behavior
      mask DialogControl BasicFipParamTab Prompt: Failure Mode Occurrence
      mask DialogControl BasicFipParam Prompt: Parameters
      mask DialogControl FailureRate_label Prompt: Failure Rate [1/h]
      mask DialogControl MaintenanceTask_label Prompt: Maintenance Task [h]
      mask DialogControl RiskTime_label Prompt: Risk time [h]
      mask DialogControl DSFipParamTab Prompt: Dependent System Information
      mask DialogControl DSFipParam Prompt: Parameters
      mask DialogControl LoadCSV Prompt: Browse
      mask DialogControl LoadCSV Callback:
      | [file,path,indx] = uigetfile('*.csv');
      | try
      |     set_param(gcb, 'File', append(path,file));
      |     file = fopen(append(path,file));
      | 
      |     fips = {};
      |     cutsets = {};
      | 
      |     line = fgetl(file);
      |     while ischar(line)
      |         disp(join([' > Processing: ',line]));
      |         splitString = split(line, ';');
      |         if isequal(splitString{1}, 'Cut set')
      |             disp('   > Found Cut set');
      |             cs = splitString(2:end-1);
      |             disp(cs);
      |             cutsets{end+1} = cs';
      |         else
      |             disp('   > Found FIP');
      |             if ~isequal("h", splitString(7))
      |                 disp('no time format except hour is supported');
      |             end
      |             fip = {};
      |             fip.id = splitString(1);
      |             fip.path = splitString(3);
      |             fip.rate = splitString(4);
      |             fip.checkInterval = splitString(6);
      |             disp(fip);
      |             fips{end+1} = fip;
      |         end
      |         line = fgetl(file);
      |     end
      | 
      |     fclose(file);
      | 
      |     DSF = {};
      |     DSF.fips = fips;
      |     DSF.cutsets = cutsets;
      | 
      |     VarCSText = jsonencode(DSF);
      |     set_param(gcb, 'DSFjson', VarCSText);
      | catch
      | end
  Out1 : Outport
  wires:
  In1/1 -> Permanently Blocked True/1(In1)
  Commit Any Bool/1(Out1) -> Out1/1
  Permanently Blocked False/1(Out1) -> Commit Any Bool/1(In1)
  Permanently Blocked True/1(Out1) -> Permanently Blocked False/1(In1)
